simulink model "TEORIA_drone_C_NL_plant_D_control"  (R2020a)
settings: Solver=FixedStepAuto  StartTime=0.0  StopTime=100  FixedStep=0.01  RelTol=1e-3
values from neighbouring files (symbols this model uses):
  Ts = 0.005    [workspaceForDrone3DAnimation.mat]    (also in workspaceForDrone3DAnimation1.mat; workspaceForDrone3DAnimation2.mat)
libraries: slctrlblks x5, simulink x4, simulink_extras x1, aerolibanimutils x1
settings Model: Creator=augus  LastModifiedBy=augus
settings DataIOCC: SaveOutput=off

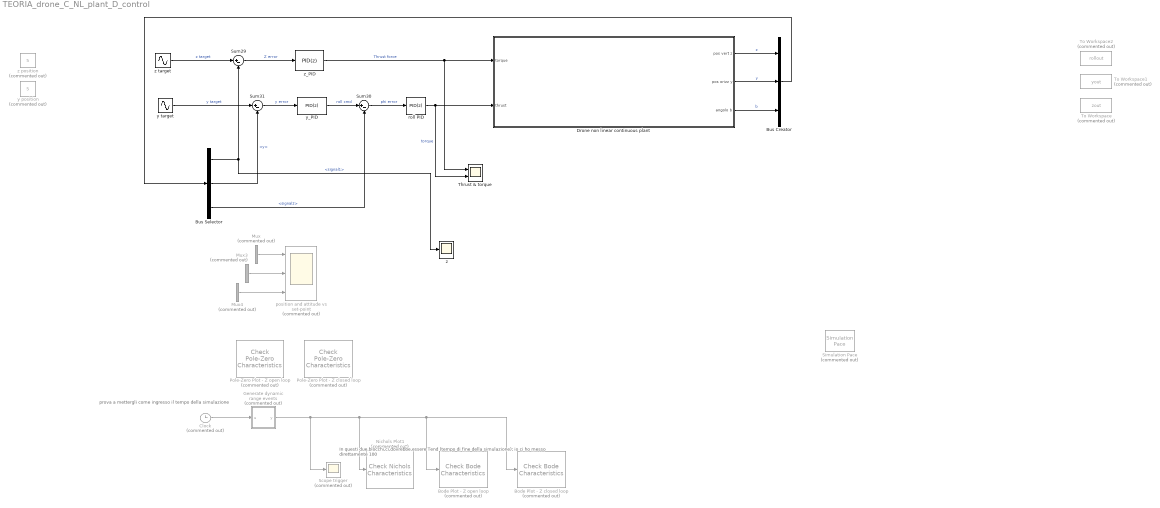
== system TEORIA_drone_C_NL_plant_D_control ==
  note: In questi due blocchi ci dovrebbe essere Tend (tempo di fine della simulazione); io ci ho messo direttamente 100
  note: prova a mettergli come ingresso il tempo della simulazione
  Bode Plot - Z closed loop : slctrlblks/Model Verification/Check Bode  Characteristics  Commented=on  InstantiateOnLoad=on  SaveOperatingPoints=off  LinearizationIOs={'/Non-linear_continuous_drone_plant', 2, 'out', 'on', '';'/z target', 1, 'in', 'off', ''}  LinearizeAt=ExternalTrigger  SnapshotTimes=[0]  TriggerType=rising  SampleTime=auto  RateConversionMethod=zoh  PreWarpFreq=10  UseExactDelayModel=off  UseFullBlockNameLabels=off  UseBusSignalLabels=off  enabled=on  stopWhenAssertionFail=off  export=off  ViewDlgPos=[985 374.6 509.6 389.6]  OpenViewOnLoad=off  LaunchViewOnOpen=off  FrequencyUnits=rad/s  MagnitudeUnits=dB  PhaseUnits=deg  TimeUnits=seconds  EnableUpperBound=off  UpperBoundFrequencies=[]  UpperBoundMagnitudes=[]  EnableLowerBound=off  LowerBoundFrequencies=[]  LowerBoundMagnitudes=[]
      settings: SaveToWorkspace=on  SaveName=sys_bode_Z_closedLoop
  Bode Plot - Z open loop : slctrlblks/Model Verification/Check Bode  Characteristics  Commented=on  InstantiateOnLoad=on  SaveOperatingPoints=off  LinearizationIOs={'/z_PID', 1, 'in', 'off', '';'/Non-linear_continuous_drone_plant', 2, 'out', 'on', ''}  LinearizeAt=ExternalTrigger  SnapshotTimes=[0]  TriggerType=rising  SampleTime=auto  RateConversionMethod=zoh  PreWarpFreq=10  UseExactDelayModel=off  UseFullBlockNameLabels=off  UseBusSignalLabels=off  enabled=on  stopWhenAssertionFail=off  export=off  ViewDlgPos=[309.8 369.8 509.6 389.6]  OpenViewOnLoad=off  LaunchViewOnOpen=off  FrequencyUnits=rad/s  MagnitudeUnits=dB  PhaseUnits=deg  TimeUnits=seconds  EnableUpperBound=off  UpperBoundFrequencies=[]  UpperBoundMagnitudes=[]  EnableLowerBound=off  LowerBoundFrequencies=[]  LowerBoundMagnitudes=[]
      settings: SaveToWorkspace=on  SaveName=sys_bode_Z_openLoop
  Bus Creator : BusCreator  Inputs=3
  Bus Selector : BusSelector  OutputSignals=signal1,y,signal2
  Clock : Clock  Commented=on
  Drone non linear continuous plant : Subsystem
  Generate dynamic range events : Subsystem  Commented=on  mask(Dynamic Range Trigger Generator){UB=100*( (0.1:0.1:0.9)+0.01 )', LB=100*( (0.1:0.1:0.9)-0.01)'}
      mask prompts: UB "Signal upper bound"; LB "Signal lower bound"
      mask help: Generates trigger events when a signal enters and exits a dynamic range. When the signal enters the dynamic range a rising edge event is fired, a falling edge event is fired when the signal leaves the dynamic range.
      mask init:
      | if length(UB) ~= length(LB)
      | 	error('The upper and lower bound settling time values must be the same.')
      | end
      mask Help:
      | <p>
      | The dynamic range trigger generator outputs trigger events when a signal enters and exits a
      | dynamic range. A rising edge event is fired when the signal enters the dynamic range specified
      | by the block parameters. A falling edge event is fired when the signal exits the dynamic range
      | specified by the block parameters.
      | </p>
      | 
      | <p>
      | Mask variables:
      | </p>
      | <ul>
      | <li> Signal upper bound - Upper limits for the signal dynamic range.  This is a vector. </li>
      | <li> Signal lower bound - Lower limits for the signal dynamic range.  This is a vector. </li>
      | </ul>
  Mux : Mux  Commented=on  Inputs=2
  Mux3 : Mux  Commented=on  Inputs=2
  Mux4 : Mux  Commented=on  Inputs=2
  Nichols Plot1 : slctrlblks/Model Verification/Check Nichols Characteristics  Commented=on  InstantiateOnLoad=on  SaveOperatingPoints=off  LinearizationIOs={'/Velocity Controller ', 1, 'outin', 'on', ''}  LinearizeAt=ExternalTrigger  SnapshotTimes=0:10:100  TriggerType=rising  ZeroCross=off  SampleTime=auto  RateConversionMethod=zoh  PreWarpFreq=10  UseExactDelayModel=off  UseFullBlockNameLabels=off  UseBusSignalLabels=off  enabled=on  stopWhenAssertionFail=off  export=off  ViewDlgPos=[583 148 510 390]  LaunchViewOnOpen=off  OpenViewOnLoad=off  FrequencyUnits=rad/s  MagnitudeUnits=dB  PhaseUnits=deg  TimeUnits=seconds  EnableMargins=off  GainMargin=[]  PhaseMargin=[]  EnableGainPhaseBound=off  GainPhaseBoundType={'upper'}  OLPhases=[]  OLGains=[]  EnableCLPeakGain=off  CLPeakGain=[]  FeedbackSign=+1
      settings: SourceProductBaseCode=SD  SaveToWorkspace=off  SaveName=sys
  Pole-Zero Plot - Z closed loop : slctrlblks/Model Verification/Check Pole-Zero Characteristics  Commented=on  InstantiateOnLoad=on  SaveOperatingPoints=off  LinearizationIOs={'/Non-linear_continuous_drone_plant', 2, 'out', 'on', '';'/z target', 1, 'in', 'off', ''}  LinearizeAt=SnapshotTimes  SnapshotTimes=[0]  TriggerType=rising  SampleTime=auto  RateConversionMethod=zoh  PreWarpFreq=10  UseExactDelayModel=off  UseFullBlockNameLabels=off  UseBusSignalLabels=off  enabled=on  stopWhenAssertionFail=off  export=off  ViewDlgPos=[734.6 74.6 509.6 389.6]  LaunchViewOnOpen=off  OpenViewOnLoad=off  FrequencyUnits=rad/s  MagnitudeUnits=dB  PhaseUnits=deg  TimeUnits=seconds  EnableSettlingTime=off  SettlingTime=[]  EnablePercentOvershoot=off  PercentOvershoot=[]  EnableDampingRatio=off  DampingRatio=[]  EnableNaturalFrequency=off  NaturalFrequencyBound=>=  NaturalFrequency=[]
      settings: SourceProductBaseCode=SD  SaveToWorkspace=on  SaveName=sys_polesZeroes_Z_closedLoop
  Pole-Zero Plot - Z open loop : slctrlblks/Model Verification/Check Pole-Zero Characteristics  Commented=on  InstantiateOnLoad=on  SaveOperatingPoints=off  LinearizationIOs={'/z_PID', 1, 'in', 'off', '';'/Non-linear_continuous_drone_plant', 2, 'out', 'on', ''}  LinearizeAt=SnapshotTimes  SnapshotTimes=[0]  TriggerType=rising  SampleTime=auto  RateConversionMethod=zoh  PreWarpFreq=10  UseExactDelayModel=off  UseFullBlockNameLabels=off  UseBusSignalLabels=off  enabled=on  stopWhenAssertionFail=off  export=off  ViewDlgPos=[128.2 81.8 509.6 389.6]  LaunchViewOnOpen=off  OpenViewOnLoad=off  FrequencyUnits=rad/s  MagnitudeUnits=dB  PhaseUnits=deg  TimeUnits=seconds  EnableSettlingTime=off  SettlingTime=[]  EnablePercentOvershoot=off  PercentOvershoot=[]  EnableDampingRatio=off  DampingRatio=[]  EnableNaturalFrequency=off  NaturalFrequencyBound=>=  NaturalFrequency=[]
      settings: SourceProductBaseCode=SD  SaveToWorkspace=on  SaveName=sys_polesZeroes_Z_openLoop
  Scope trigger : Scope  Commented=on
  Simulation Pace : aerolibanimutils/Simulation Pace  Commented=on  SimulationPace=1  SleepMode=MATLAB Thread  OutputPaceError=off  SampleTime=Ts
      settings: AttributesFormatString=%<SimulationPace> sec/sec
  Sum29 : Sum  Inputs=|+-
  Sum30 : Sum  Inputs=|+-
  Sum31 : Sum  Inputs=|+-
  Thrust & torque : Scope  NumInputPorts=2
  To Workspace : ToWorkspace  Commented=on  VariableName=zout  SampleTime=-1
  To Workspace1 : ToWorkspace  Commented=on  VariableName=yout  SampleTime=-1
  To Workspace2 : ToWorkspace  Commented=on  VariableName=rollout  SampleTime=-1
  position and attitude vs set-point : Scope  Commented=on  NumInputPorts=3
  roll PID : simulink/Continuous/PID Controller  Controller=PID  Form=Parallel  TimeDomain=Discrete-time  UseExternalTs=off  SampleTime=0.01  IntegratorMethod=Forward Euler  FilterMethod=Forward Euler  ControllerParametersSource=internal  P=0.6  I=0  D=0.7  UseFilter=on  N=100  TunerSelectOption=Transfer Function Based (PID Tuner App)  InitialConditionSource=internal  InitialConditionForIntegrator=0  InitialConditionForFilter=0  DifferentiatorICPrevScaledInput=0  ExternalReset=none  TrackingMode=off  Kt=1  LimitOutput=off  UpperSaturationLimit=inf  LowerSaturationLimit=-inf  LinearizeAsGain=on  AntiWindupMode=none  Kb=1  POutMin=[]  POutMax=[]  IOutMin=[]  IOutMax=[]  DOutMin=[]  DOutMax=[]  NOutMin=[]  NOutMax=[]  SumOutMin=[]  SumOutMax=[]  SaturationOutMin=[]  SaturationOutMax=[]  PParamMin=[]  PParamMax=[]  IParamMin=[]  IParamMax=[]  DParamMin=[]  DParamMax=[]  NParamMin=[]  NParamMax=[]  KbParamMin=[]  KbParamMax=[]  KtParamMin=[]  KtParamMax=[]  KbOutMin=[]  KbOutMax=[]  KtOutMin=[]  KtOutMax=[]  IntegratorOutMin=[]  IntegratorOutMax=[]  FilterOutMin=[]  FilterOutMax=[]  SumI1OutMin=[]  SumI1OutMax=[]  SumI2OutMin=[]  SumI2OutMax=[]  SumI3OutMin=[]  SumI3OutMax=[]  SumI4OutMin=[]  SumI4OutMax=[]  SumDOutMin=[]  SumDOutMax=[]  DifferentiatorOutMin=[]  DifferentiatorOutMax=[]  FilterDiffOutCoefMin=[]  FilterDiffOutCoefMax=[]  ReciprocalOutMin=[]  ReciprocalOutMax=[]  SumDenOutMin=[]  SumDenOutMax=[]  SumNumOutMin=[]  SumNumOutMax=[]  DivideOutMin=[]  DivideOutMax=[]  UdiffTsProdOutMin=[]  UdiffTsProdOutMax=[]  NTsProdOutMin=[]  NTsProdOutMax=[]  UintegralTsProdOutMin=[]  UintegralTsProdOutMax=[]  UngainTsProdOutMin=[]  UngainTsProdOutMax=[]  IntegratorContinuousStateAttributes=''  IntegratorStateMustResolveToSignalObject=off  IntegratorRTWStateStorageClass=Auto  FilterContinuousStateAttributes=''  FilterStateMustResolveToSignalObject=off  FilterRTWStateStorageClass=Auto  ParallelPVariant=InternalParameters  IdealPVariant=Disabled  IVariant=InternalParameters  DVariant=InternalParameters  IntegratorVariant=Discrete  SatVariant=Disabled  AWVariant=Passthrough  PCopyVariant=Disabled  TRVariant=Disabled  FdbkBlocksVariant=Forward  IdealPFdbkVariant=Disabled  SatFdbkVariant=Disabled  DerivativeFilterVariant=ForwardEulerFilter  NVariant=InternalParameters  NCopyVariant=Disabled  FilterICVariant=InternalICsFilter  IntegratorICVariant=InternalICs  ExternalResetVariant=Disabled  TRSumVariant=Passthrough  SumFdbkVariant=Disabled  SumVariant=Sum_PID  TsampFilterVariant=InternalTs  TsampNgainVariant=Passthrough  TsampIntegralVariant=Passthrough
  y position : Constant  Commented=on  Value=5
  y target : Sin  Amplitude=2  Frequency=0.25  SampleTime=0
  y_PID : simulink/Continuous/PID Controller  Controller=PID  Form=Parallel  TimeDomain=Discrete-time  UseExternalTs=off  SampleTime=0.01  IntegratorMethod=Forward Euler  FilterMethod=Forward Euler  ControllerParametersSource=internal  P=0.50  I=0  D=0.4  UseFilter=on  N=100  TunerSelectOption=Transfer Function Based (PID Tuner App)  InitialConditionSource=internal  InitialConditionForIntegrator=0  InitialConditionForFilter=0  DifferentiatorICPrevScaledInput=0  ExternalReset=none  TrackingMode=off  Kt=1  LimitOutput=on  UpperSaturationLimit=0.52  LowerSaturationLimit=-0.52  LinearizeAsGain=on  AntiWindupMode=none  Kb=1  POutMin=[]  POutMax=[]  IOutMin=[]  IOutMax=[]  DOutMin=[]  DOutMax=[]  NOutMin=[]  NOutMax=[]  SumOutMin=[]  SumOutMax=[]  SaturationOutMin=[]  SaturationOutMax=[]  PParamMin=[]  PParamMax=[]  IParamMin=[]  IParamMax=[]  DParamMin=[]  DParamMax=[]  NParamMin=[]  NParamMax=[]  KbParamMin=[]  KbParamMax=[]  KtParamMin=[]  KtParamMax=[]  KbOutMin=[]  KbOutMax=[]  KtOutMin=[]  KtOutMax=[]  IntegratorOutMin=[]  IntegratorOutMax=[]  FilterOutMin=[]  FilterOutMax=[]  SumI1OutMin=[]  SumI1OutMax=[]  SumI2OutMin=[]  SumI2OutMax=[]  SumI3OutMin=[]  SumI3OutMax=[]  SumI4OutMin=[]  SumI4OutMax=[]  SumDOutMin=[]  SumDOutMax=[]  DifferentiatorOutMin=[]  DifferentiatorOutMax=[]  FilterDiffOutCoefMin=[]  FilterDiffOutCoefMax=[]  ReciprocalOutMin=[]  ReciprocalOutMax=[]  SumDenOutMin=[]  SumDenOutMax=[]  SumNumOutMin=[]  SumNumOutMax=[]  DivideOutMin=[]  DivideOutMax=[]  UdiffTsProdOutMin=[]  UdiffTsProdOutMax=[]  NTsProdOutMin=[]  NTsProdOutMax=[]  UintegralTsProdOutMin=[]  UintegralTsProdOutMax=[]  UngainTsProdOutMin=[]  UngainTsProdOutMax=[]  IntegratorContinuousStateAttributes=''  IntegratorStateMustResolveToSignalObject=off  IntegratorRTWStateStorageClass=Auto  FilterContinuousStateAttributes=''  FilterStateMustResolveToSignalObject=off  FilterRTWStateStorageClass=Auto  ParallelPVariant=InternalParameters  IdealPVariant=Disabled  IVariant=InternalParameters  DVariant=InternalParameters  IntegratorVariant=Discrete  SatVariant=Enabled  AWVariant=Passthrough  PCopyVariant=Disabled  TRVariant=Disabled  FdbkBlocksVariant=Forward  IdealPFdbkVariant=Disabled  SatFdbkVariant=Disabled  DerivativeFilterVariant=ForwardEulerFilter  NVariant=InternalParameters  NCopyVariant=Disabled  FilterICVariant=InternalICsFilter  IntegratorICVariant=InternalICs  ExternalResetVariant=Disabled  TRSumVariant=Passthrough  SumFdbkVariant=Disabled  SumVariant=Sum_PID  TsampFilterVariant=InternalTs  TsampNgainVariant=Passthrough  TsampIntegralVariant=Passthrough
  z : Scope
  z position : Constant  Commented=on  Value=5
  z target : Sin  Amplitude=3  Frequency=0.5  SampleTime=0
  z_PID : simulink/Continuous/PID Controller  Controller=PID  Form=Parallel  TimeDomain=Discrete-time  UseExternalTs=off  SampleTime=0.01  IntegratorMethod=Forward Euler  FilterMethod=Forward Euler  ControllerParametersSource=internal  P=0.65  I=0.3  D=0.35  UseFilter=on  N=100  TunerSelectOption=Transfer Function Based (PID Tuner App)  InitialConditionSource=internal  InitialConditionForIntegrator=0  InitialConditionForFilter=0  DifferentiatorICPrevScaledInput=0  ExternalReset=none  TrackingMode=off  Kt=1  LimitOutput=on  UpperSaturationLimit=30  LowerSaturationLimit=0  LinearizeAsGain=on  AntiWindupMode=none  Kb=1  POutMin=[]  POutMax=[]  IOutMin=[]  IOutMax=[]  DOutMin=[]  DOutMax=[]  NOutMin=[]  NOutMax=[]  SumOutMin=[]  SumOutMax=[]  SaturationOutMin=[]  SaturationOutMax=[]  PParamMin=[]  PParamMax=[]  IParamMin=[]  IParamMax=[]  DParamMin=[]  DParamMax=[]  NParamMin=[]  NParamMax=[]  KbParamMin=[]  KbParamMax=[]  KtParamMin=[]  KtParamMax=[]  KbOutMin=[]  KbOutMax=[]  KtOutMin=[]  KtOutMax=[]  IntegratorOutMin=[]  IntegratorOutMax=[]  FilterOutMin=[]  FilterOutMax=[]  SumI1OutMin=[]  SumI1OutMax=[]  SumI2OutMin=[]  SumI2OutMax=[]  SumI3OutMin=[]  SumI3OutMax=[]  SumI4OutMin=[]  SumI4OutMax=[]  SumDOutMin=[]  SumDOutMax=[]  DifferentiatorOutMin=[]  DifferentiatorOutMax=[]  FilterDiffOutCoefMin=[]  FilterDiffOutCoefMax=[]  ReciprocalOutMin=[]  ReciprocalOutMax=[]  SumDenOutMin=[]  SumDenOutMax=[]  SumNumOutMin=[]  SumNumOutMax=[]  DivideOutMin=[]  DivideOutMax=[]  UdiffTsProdOutMin=[]  UdiffTsProdOutMax=[]  NTsProdOutMin=[]  NTsProdOutMax=[]  UintegralTsProdOutMin=[]  UintegralTsProdOutMax=[]  UngainTsProdOutMin=[]  UngainTsProdOutMax=[]  IntegratorContinuousStateAttributes=''  IntegratorStateMustResolveToSignalObject=off  IntegratorRTWStateStorageClass=Auto  FilterContinuousStateAttributes=''  FilterStateMustResolveToSignalObject=off  FilterRTWStateStorageClass=Auto  ParallelPVariant=InternalParameters  IdealPVariant=Disabled  IVariant=InternalParameters  DVariant=InternalParameters  IntegratorVariant=Discrete  SatVariant=Enabled  AWVariant=Passthrough  PCopyVariant=Disabled  TRVariant=Disabled  FdbkBlocksVariant=Forward  IdealPFdbkVariant=Disabled  SatFdbkVariant=Disabled  DerivativeFilterVariant=ForwardEulerFilter  NVariant=InternalParameters  NCopyVariant=Disabled  FilterICVariant=InternalICsFilter  IntegratorICVariant=InternalICs  ExternalResetVariant=Disabled  TRSumVariant=Passthrough  SumFdbkVariant=Disabled  SumVariant=Sum_PID  TsampFilterVariant=InternalTs  TsampNgainVariant=Passthrough  TsampIntegralVariant=Passthrough
  wires:
  z target/1 -> Sum29/1  "z target"
  z_PID/1 -> Drone non linear continuous plant/1(torque), Thrust & torque/1  "Thrust force"
  Sum29/1 -> z_PID/1  "Z error"
  Sum30/1 -> roll PID/1  "phi error"
  y target/1 -> Sum31/1  "y target"
  Sum31/1 -> y_PID/1  "y error"
  y_PID/1 -> Sum30/1  "roll cmd"
  roll PID/1 -> Thrust & torque/2, Drone non linear continuous plant/2(thrust)  "torque"
  Mux/1 -> position and attitude vs set-point/1
  Mux3/1 -> position and attitude vs set-point/2
  Mux4/1 -> position and attitude vs set-point/3
  Generate dynamic range events/1(y) -> Bode Plot - Z closed loop/1, Bode Plot - Z open loop/1, Nichols Plot1/1, Scope trigger/1
  Clock/1 -> Generate dynamic range events/1(u)
  Drone non linear continuous plant/1(pos vert z) -> Bus Creator/1  "z"
  Drone non linear continuous plant/2(pos orizz y) -> Bus Creator/2  "y"
  Drone non linear continuous plant/3(angolo b) -> Bus Creator/3  "b"
  Bus Creator/1 -> Bus Selector/1
  Bus Selector/2 -> Sum31/2  "<y>"
  Bus Selector/1 -> z/1, Sum29/2  "<signal1>"
  Bus Selector/3 -> Sum30/2  "<signal2>"

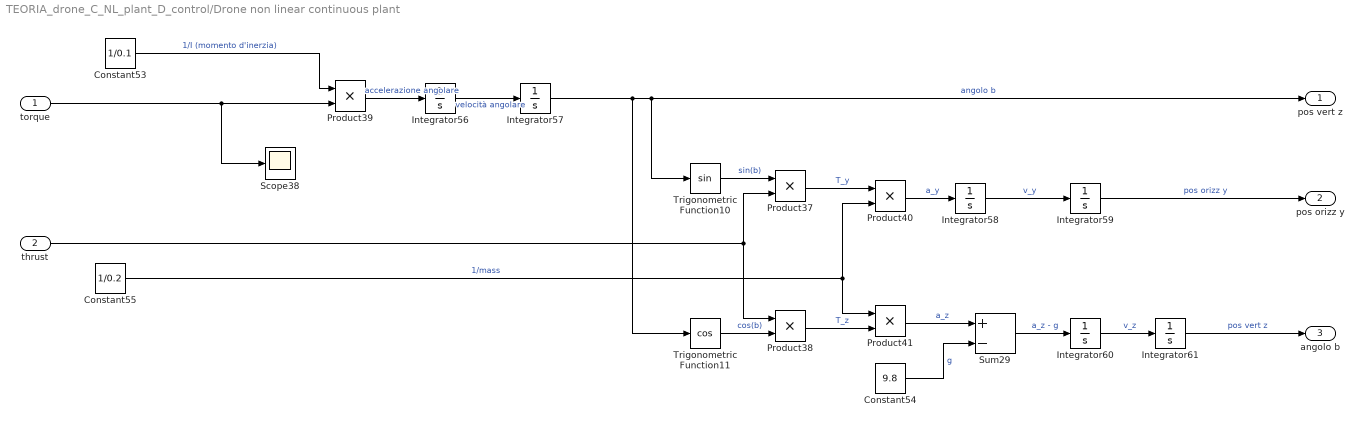
== system TEORIA_drone_C_NL_plant_D_control/Drone non linear continuous plant ==
  torque : Inport
  thrust : Inport  Port=2
  Constant53 : Constant  Value=1/0.1
  Constant54 : Constant  Value=9.8
  Constant55 : Constant  Value=1/0.2
  Integrator{56..61} (6 alike) : Integrator
  Product{37..41} (5 alike) : Product
  Scope38 : Scope
  Sum29 : Sum  Inputs=+-
  Trigonometric Function10 : Trigonometry
  Trigonometric Function11 : Trigonometry  Operator=cos
  pos vert z : Outport
  pos orizz y : Outport  Port=2
  angolo b : Outport  Port=3
  wires:
  Integrator60/1 -> Integrator61/1  "v_z"
  Integrator57/1 -> pos vert z/1, Trigonometric Function10/1, Trigonometric Function11/1  "angolo b"
  Constant55/1 -> Product41/1, Product40/2  "1/mass"
  torque/1 -> Product39/2, Scope38/1
  Product38/1 -> Product41/2  "T_z"
  thrust/1 -> Product38/1, Product37/2
  Constant53/1 -> Product39/1  "1/I (momento d'inerzia)"
  Product39/1 -> Integrator56/1  "accelerazione angolare"
  Integrator56/1 -> Integrator57/1  "velocità angolare"
  Product37/1 -> Product40/1  "T_y"
  Trigonometric Function11/1 -> Product38/2  "cos(b)"
  Product41/1 -> Sum29/1  "a_z"
  Integrator58/1 -> Integrator59/1  "v_y"
  Trigonometric Function10/1 -> Product37/1  "sin(b)"
  Sum29/1 -> Integrator60/1  "a_z - g"
  Product40/1 -> Integrator58/1  "a_y"
  Constant54/1 -> Sum29/2  "g"
  Integrator59/1 -> pos orizz y/1  "pos orizz y"
  Integrator61/1 -> angolo b/1  "pos vert z"

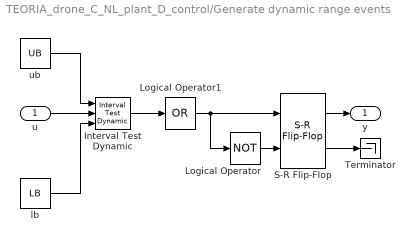
== system TEORIA_drone_C_NL_plant_D_control/Generate dynamic range events ==
  u : Inport
  Interval Test Dynamic : simulink/Logic and Bit Operations/Interval Test Dynamic  IntervalClosedRight=on  IntervalClosedLeft=on  OutDataTypeStr=boolean
      settings: SourceProductBaseCode=SL
  Logical Operator : Logic  Operator=NOT  AllPortsSameDT=off  OutDataTypeStr=boolean
  Logical Operator1 : Logic  Operator=OR  Inputs=1  AllPortsSameDT=off  OutDataTypeStr=boolean
  S-R Flip-Flop : simulink_extras/Flip Flops/S-R Flip-Flop  initial_condition=0
  Terminator : Terminator
  lb : Constant  Value=LB
  ub : Constant  Value=UB
  y : Outport  VectorParamsAs1DForOutWhenUnconnected=off
  wires:
  S-R Flip-Flop/1 -> y/1
  u/1 -> Interval Test Dynamic/2
  Logical Operator1/1 -> Logical Operator/1, S-R Flip-Flop/1
  lb/1 -> Interval Test Dynamic/3
  ub/1 -> Interval Test Dynamic/1
  Interval Test Dynamic/1 -> Logical Operator1/1
  S-R Flip-Flop/2 -> Terminator/1
  Logical Operator/1 -> S-R Flip-Flop/2
